simulink model "disc"  (R2022a)
settings: Solver=FixedStepDiscrete  StartTime=0.0  StopTime=30  FixedStep=delta_time  RelTol=1e-3
libraries: cstblocks x3
settings Model: Creator=phcs  LastModifiedBy=phcs

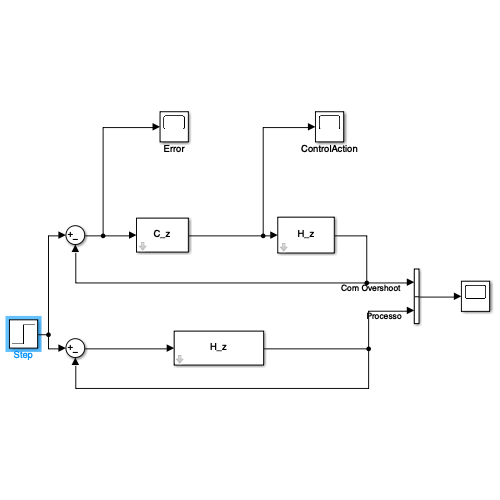
[thumbnail: Simulink's stored preview of the top-level diagram]
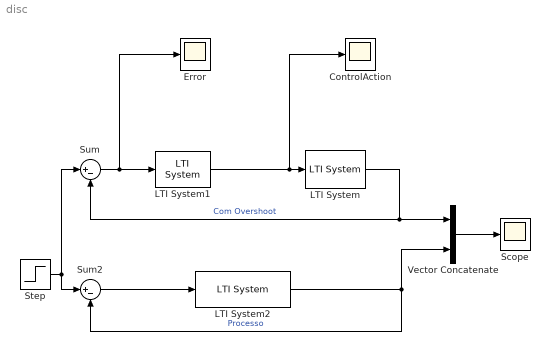
== system disc ==
  ControlAction : Scope
  Error : Scope
  LTI System : cstblocks/LTI System  sys=H_z  IC=[]
  LTI System1 : cstblocks/LTI System  sys=C_z  IC=[]
  LTI System2 : cstblocks/LTI System  sys=H_z  IC=[]
  Scope : Scope
  Step : Step  Time=0  SampleTime=0
  Sum : Sum  Inputs=|+-
  Sum2 : Sum  Inputs=|+-
  Vector Concatenate : Concatenate
  wires:
  LTI System/1 -> Vector Concatenate/1, Sum/2  "Com Overshoot"
  Vector Concatenate/1 -> Scope/1
  Sum2/1 -> LTI System2/1
  LTI System2/1 -> Vector Concatenate/2, Sum2/2  "Processo"
  Step/1 -> Sum2/1, Sum/1
  LTI System1/1 -> ControlAction/1, LTI System/1
  Sum/1 -> Error/1, LTI System1/1
